simulink model "simulink_model"  (R2017b)
settings: Solver=VariableStepAuto  StartTime=0.0  StopTime=10.0  RelTol=1e-3
values from neighbouring files (symbols this model uses):
  l = 1    [pendulum_parameters.m]
  m = 1    [pendulum_parameters.m]
  M = 1    [pendulum_parameters.m]
  omega0 = 0    [pendulum_parameters.m]
  theta0 = pi/2    (= 1.57079632679)    [pendulum_parameters.m]
  v0 = 0    [pendulum_parameters.m]
  x0 = 0    [pendulum_parameters.m]
settings Model: Creator=alexe  LastModifiedBy=alexe

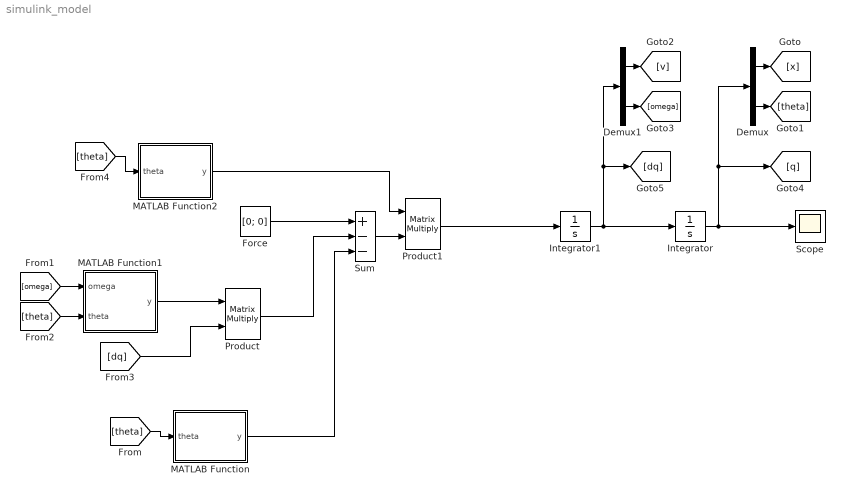
== system simulink_model ==
  Demux : Demux  Outputs=2
  Demux1 : Demux  Outputs=2
  Force : Constant  Value=[0; 0]
  Integrator : Integrator  InitialCondition=[x0; theta0]
  Integrator1 : Integrator  InitialCondition=[v0; omega0]
  MATLAB Function : MATLAB Function  TreatAsAtomicUnit=on
  MATLAB Function1 : MATLAB Function  TreatAsAtomicUnit=on
  MATLAB Function2 : MATLAB Function  TreatAsAtomicUnit=on
  Product : Product  Multiplication=Matrix(*)
  Product1 : Product  Multiplication=Matrix(*)
  Scope : Scope
  Sum : Sum  Inputs=+--
  wires:
  Integrator1/1 -> [dq], Demux1/1, Integrator/1
  Integrator/1 -> [q], Demux/1, Scope/1
  Demux/1 -> [x]
  Demux/2 -> [theta]
  Demux1/2 -> [omega]
  Demux1/1 -> [v]
  [theta] -> MATLAB Function/1(theta)
  [omega] -> MATLAB Function1/1(omega)
  [theta] -> MATLAB Function1/2(theta)
  MATLAB Function1/1(y) -> Product/1
  [dq] -> Product/2
  Force/1 -> Sum/1
  Product/1 -> Sum/2
  MATLAB Function/1(y) -> Sum/3
  [theta] -> MATLAB Function2/1(theta)
  Sum/1 -> Product1/2
  MATLAB Function2/1(y) -> Product1/1
  Product1/1 -> Integrator1/1

== matlab function simulink_model/MATLAB Function1 ==
  data: omega input; theta input; y output; m parameter; l parameter
function y = C(omega, theta, m, l)

y = [m*l*omega*sin(theta) 0; 0 0];

== matlab function simulink_model/MATLAB Function ==
  data: theta input; y output; g parameter
function y = g(theta, g)

y = [0; -g*sin(theta)];

== matlab function simulink_model/MATLAB Function2 ==
  data: theta input; y output; M parameter; m parameter; l parameter
function y = inv_M(theta, M, m, l)
temp = [M+m -m*l*cos(theta); -cos(theta) l]
y = inv(temp);
